simulink model "No_3_PID_Controller_Simulink"  (R2013b)
settings: Solver=ode4  StartTime=0  StopTime=30  FixedStep=0.001  RelTol=1e-3
settings Model: Creator=ZEROO  LastModifiedBy=ZEROO
settings GRTTargetCC: LogVarNameModifier=none

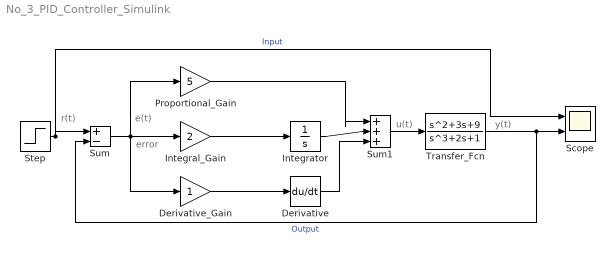
== system No_3_PID_Controller_Simulink ==
  note: y(t)
  note: u(t)
  note: error
  note: r(t)
  note: e(t)
  Derivative : Derivative
  Derivative_Gain : Gain
  Integral_Gain : Gain  Gain=2
  Integrator : Integrator
  Proportional_Gain : Gain  Gain=5
  Scope : Scope  NumInputPorts=2
      settings: ShowLegends=on  TimeRange=30  YMin=-0.2~-0.2  YMax=1.2~1.2  SaveName=Data
  Step : Step  SampleTime=0
  Sum : Sum  Inputs=|+-
  Sum1 : Sum  Inputs=|+++
  Transfer_Fcn : TransferFcn  Numerator=[1 3 9]  Denominator=[1 0 2 1]
  wires:
  Step/1 -> Scope/1, Sum/1  "Input"
  Transfer_Fcn/1 -> Scope/2, Sum/2  "Output"
  Sum/1 -> Integral_Gain/1, Proportional_Gain/1, Derivative_Gain/1
  Integral_Gain/1 -> Integrator/1
  Derivative_Gain/1 -> Derivative/1
  Sum1/1 -> Transfer_Fcn/1
  Proportional_Gain/1 -> Sum1/1
  Integrator/1 -> Sum1/2
  Derivative/1 -> Sum1/3
